simulink model "threeQ_cascaded_relays_real_2024a"  (R2024a)
settings: Solver=VariableStepAuto  StartTime=0.0  StopTime=15  RelTol=1e-3
libraries: spsThreePhaseSeriesRLCLoadLib x2, spsThreePhaseVIMeasurementLib x2, spsThreePhaseBreakerLib x2, spsThreePhaseFaultLib x2, spsDistributedParametersLineLib x1, spsThreePhaseSourceLib x1, spspowerguiLib x1
settings Model: SimulationMode=accelerator  Creator=Carnival  LastModifiedBy=user

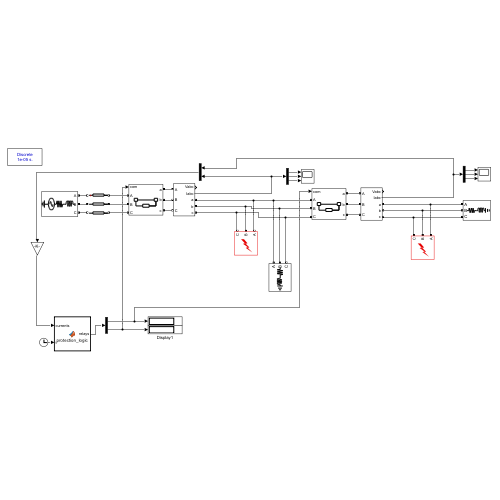
[thumbnail: Simulink's stored preview of the top-level diagram]
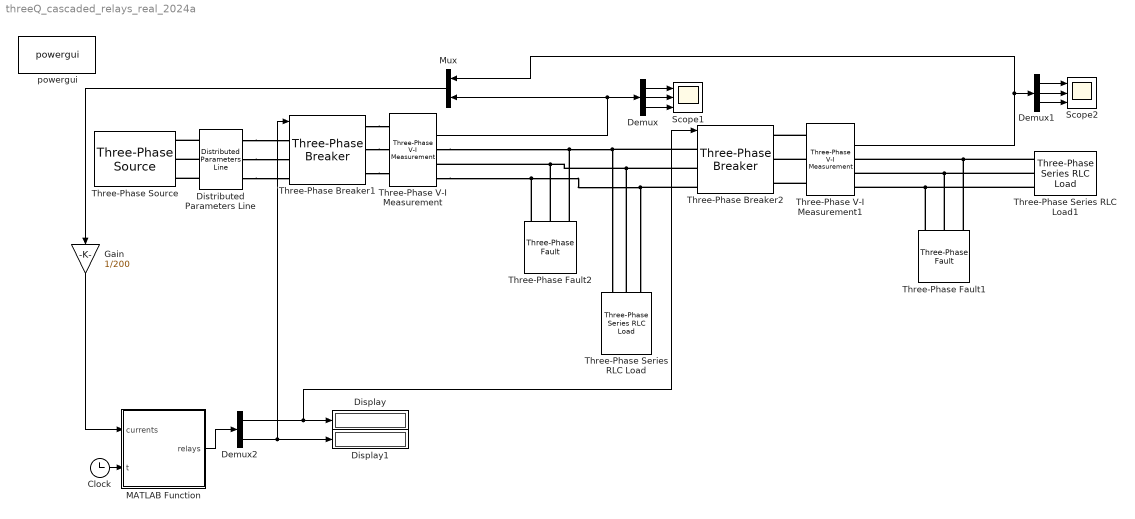
== system threeQ_cascaded_relays_real_2024a ==
  Clock : Clock
  Demux : Demux  Outputs=3
  Demux1 : Demux  Outputs=3
  Demux2 : Demux  Outputs=2
  Display : Display
  Display1 : Display
  Distributed Parameters Line : spsDistributedParametersLineLib/Distributed Parameters Line  Phases=3  Length=15  Frequency=50  Resistance=[0.6273 0.8864]  Inductance="[0.9337e-3  4.1264e-3]"  Capacitance=[12.74e-9 7.751e-9]  x1=[-9e-05 5.02208795910123e-09 1588.76236265853 -8067.37575327395;-8e-05 4.99086976271208e-09 1614.09888914727 -8062.34470644657;-7e-05 4.95960230845327e-09 1639.41948513161 -8057.23408753183;-6e-05 4.92828590492195e-09 1664.72390070749 -8052.04394696949;-5e-05 4.89692086119837e-09 1690.01188613055 -8046.77433598413;-4e-05 4.86550748684287e-09 1715.28319181857 -8041.42530658469;-3e-05 4.83404609189275e-09 1740.53756835399 -8035.99691156393;-2e-05 4.80253698685929e-09 1765.77476648628 -8030.48920449791;-1e-05 4.77098048272463e-09 1790.9945371345 -8024.90223974549]  x2=[-9e-05 4.39159241008057e-08 108.20401185903 -384.846711119618;-8e-05 4.37876771750741e-08 109.412507505629 -384.504879609457;-7e-05 4.36589980826465e-08 110.61992329495 -384.159253191366;-6e-05 4.35298880935337e-08 111.826247310288 -383.809835276536;-5e-05 4.34003484819991e-08 113.03146764571 -383.456629313583;-4e-05 4.32703805265465e-08 114.23557240618 -383.099638788506;-3e-05 4.3139985509907e-08 115.438549707668 -382.738867224658;-2e-05 4.30091647190269e-08 116.640387677276 -382.374318182709;-1e-05 4.28779194450545e-08 117.841074453347 -382.005995260609]  x3=[-9e-05 2.00094431508933e-09 186.56182138791 688.697630075146;-8e-05 2.00283742250668e-09 184.397296886789 689.280331774759;-7e-05 2.00471076272724e-09 182.230952458792 689.856230555771;-6e-05 2.00656431726192e-09 180.062809484864 690.425320734294;-5e-05 2.00839806781686e-09 177.8928893637 690.987596693637;-4e-05 2.0102119962937e-09 175.721213511537 691.543052884364;-3e-05 2.01200608478969e-09 173.547803361938 692.091683824346;-2e-05 2.01378031559791e-09 171.372680365584 692.633484098817;-1e-05 2.0155346712074e-09 169.195865990061 693.168448360428]  x4=[-9e-05 -1.93383320357452e-09 -180.703878471693 -719.166809410987;-8e-05 -1.93593922240759e-09 -178.443661285832 -719.730957511193;-7e-05 -1.9380261343021e-09 -176.181682933075 -720.288002157416;-6e-05 -1.94009391866109e-09 -173.917965738234 -720.837937851849;-5e-05 -1.94214255507634e-09 -171.652532043286 -721.38075916685;-4e-05 -1.94417202332865e-09 -169.385404207145 -721.916460744991;-3e-05 -1.94618230338798e-09 -167.116604605448 -722.445037299114;-2e-05 -1.94817337541369e-09 -164.846155630331 -722.966483612381;-1e-05 -1.95014521975468e-09 -162.57407969021 -723.480794538329]  x5=8.48312350493614e-05  V1=ones(3,3)  V2=ones(3,3)  I1=ones(3,3)  I2=ones(3,3)  nHarmo=1  Measurements=None  Decoupling=off  VsMag0=0  VrMag0=0  VsAngle0=0  VrAngle0=0  IsMag0=0  IrMag0=0  IsAngle0=0  IrAngle0=0
      settings: LibrarySourceBlock=sps_lib/Power Grid Elements/Distributed Parameters Line
  Gain : Gain  Gain=1/200
  MATLAB Function : MATLAB Function  TreatAsAtomicUnit=on
  Mux : Mux  Inputs=2
  Scope1 : Scope  NumInputPorts=3
  Scope2 : Scope  NumInputPorts=3
  Three-Phase Series RLC Load : spsThreePhaseSeriesRLCLoadLib/Three-Phase Series RLC Load  LConnTagsString=A|B|C  Configuration=Y (grounded)  NominalVoltage=11000  Vabc=[1e3 1e3 1e3]  Vabcp=[1e3 1e3 1e3]  NominalFrequency=50  UnbalancedPower=off  ActivePower=2e6  InductivePower=1.2e6  CapacitivePower=0  Pabc=[10e3 9e3 11e3]  QLabc=[100 90 110]  QCabc=[100 90 110]  Pabcp=[10e3 9e3 11e3]  QLabcp=[100 90 110]  QCabcp=[100 90 110]  Measurements=None  LoadType=constant Z
  Three-Phase Series RLC Load1 : spsThreePhaseSeriesRLCLoadLib/Three-Phase Series RLC Load  LConnTagsString=A|B|C  Configuration=Y (grounded)  NominalVoltage=1100  Vabc=[1e3 1e3 1e3]  Vabcp=[1e3 1e3 1e3]  NominalFrequency=50  UnbalancedPower=off  ActivePower=2e6  InductivePower=1.2e6  CapacitivePower=0  Pabc=[10e3 9e3 11e3]  QLabc=[100 90 110]  QCabc=[100 90 110]  Pabcp=[10e3 9e3 11e3]  QLabcp=[100 90 110]  QCabcp=[100 90 110]  Measurements=None  LoadType=constant Z
  Three-Phase V-I Measurement : spsThreePhaseVIMeasurementLib/Three-Phase V-I Measurement  VoltageMeasurement=phase-to-ground  SetLabelV=off  LabelV=Vabc  Vpu=off  VpuLL=off  CurrentMeasurement=yes  SetLabelI=off  LabelI=Iabc  Ipu=off  Pbase=100e6  Vbase=500e3  OutputType=Complex  PhasorSimulation=off  PSBequivalent=0
  Three-Phase V-I Measurement1 : spsThreePhaseVIMeasurementLib/Three-Phase V-I Measurement  VoltageMeasurement=phase-to-ground  SetLabelV=off  LabelV=Vabc  Vpu=off  VpuLL=off  CurrentMeasurement=yes  SetLabelI=off  LabelI=Iabc  Ipu=off  Pbase=100e6  Vbase=500e3  OutputType=Complex  PhasorSimulation=off  PSBequivalent=0
  Three-Phase Breaker1 : spsThreePhaseBreakerLib/Three-Phase Breaker  InitialState=closed  SwitchA=on  SwitchB=on  SwitchC=on  SwitchTimes="[1/60  5/60]"  External=on  BreakerResistance=0.01  SnubberResistance=1e6  SnubberCapacitance=inf  Measurements=None
  Three-Phase Breaker2 : spsThreePhaseBreakerLib/Three-Phase Breaker  InitialState=closed  SwitchA=on  SwitchB=on  SwitchC=on  SwitchTimes="[1/60  5/60]"  External=on  BreakerResistance=0.01  SnubberResistance=1e6  SnubberCapacitance=inf  Measurements=None
  Three-Phase Fault1 : spsThreePhaseFaultLib/Three-Phase Fault  InitialStates=0  FaultA=off  FaultB=on  FaultC=on  GroundFault=on  SwitchTimes="[5  6]"  External=off  SwitchStatus=NaN  FaultResistance=0.001  GroundResistance=0.01  SnubberResistance=1e6  SnubberCapacitance=inf  Measurements=None
  Three-Phase Fault2 : spsThreePhaseFaultLib/Three-Phase Fault  InitialStates=0  FaultA=off  FaultB=on  FaultC=on  GroundFault=off  SwitchTimes="[5  6]"  External=off  SwitchStatus=NaN  FaultResistance=0.001  GroundResistance=0.01  SnubberResistance=1e6  SnubberCapacitance=inf  Measurements=None
  Three-Phase Source : spsThreePhaseSourceLib/Three-Phase Source  InternalConnection=Yg  VoltagePhases=off  Voltage=11000  PhaseAngle=0  Voltage_phases=[25e3 25e3 25e3]/sqrt(3)  PhaseAngles_phases=[0 -120 +120]  Frequency=50  NonIdealSource=on  SpecifyImpedance=off  Resistance=0.8929  Inductance=16.58e-3  ShortCircuitLevel=100e6  BaseVoltage=11000  XRratio=7  BusType=swing  Pref=10e3  Qref=0  Prefabc=[10e3, 10e3, 10e3]  Qrefabc=[0, 0, 0]  Qmin=-inf  Qmax=inf
  powergui : spspowerguiLib/powergui  Priority=1  SimulationMode=Discrete  SampleTime=1e-5  frequency=60  Iterations=50  frequencyindice=0  Pbase=100e6  ErrMax=1e-4  UnitsV=kV  UnitsW=MW  buscounter=0  FunctionMessages=off  echomessages=off  EnableUseOfTLC=off  CurrentSourceSwitches=off  DisableSnubberDevices=off  DisableRonSwitches=off  DisableVfSwitches=off  DisplayEquations=off  AutomaticDiscreteSolvers=off  SolverType=Tustin/Backward Euler (TBE)  Interpol=off  ExternalGateDelay=off  methode=off  Ts=100  x0status=blocks  SPID=on  SwTol=0  HookPort=off  NonlinearTolerance=1e-4  nMaxIteration=100  ContinueOnMaxIteration=off  RestoreLinks=warning  ResistiveCurrentMeasurement=off  Frange=[0:2:500]  Ylog=off  Xlog=on  ShowGrid=off  save=off  variable=ZData  structure=0  ZoomFFT=off  StartTime=0.0  cycles=1  DisplayStyle=1  fundamental=60  FreqAxis=off  MaxFrequency=1000  frequencyindicesteady=1  RmsSteady=1  display=off
  wires:
  Three-Phase V-I Measurement/2 -> Mux/2, Demux/1
  Three-Phase V-I Measurement1/2 -> Mux/1, Demux1/1
  Demux/1 -> Scope1/1
  Demux/2 -> Scope1/2
  Demux/3 -> Scope1/3
  Demux1/1 -> Scope2/1
  Demux1/2 -> Scope2/2
  Demux1/3 -> Scope2/3
  Clock/1 -> MATLAB Function/2(t)
  Demux2/1 -> Display/1, Three-Phase Breaker2/1
  Mux/1 -> Gain/1
  Gain/1 -> MATLAB Function/1(currents)
  MATLAB Function/1(relays) -> Demux2/1
  Demux2/2 -> Display1/1, Three-Phase Breaker1/1
  connections:
  Three-Phase Breaker1/RConn1 -- Three-Phase V-I Measurement/LConn1
  Three-Phase Breaker1/RConn2 -- Three-Phase V-I Measurement/LConn2
  Three-Phase Breaker1/RConn3 -- Three-Phase V-I Measurement/LConn3
  Three-Phase V-I Measurement/RConn1 -- Three-Phase Fault2/LConn1 -- Three-Phase Breaker2/LConn1 -- Three-Phase Series RLC Load/LConn1
  Three-Phase Series RLC Load/LConn2 -- Three-Phase V-I Measurement/RConn2 -- Three-Phase Fault2/LConn2 -- Three-Phase Breaker2/LConn2
  Three-Phase V-I Measurement/RConn3 -- Three-Phase Fault2/LConn3 -- Three-Phase Breaker2/LConn3 -- Three-Phase Series RLC Load/LConn3
  Three-Phase V-I Measurement1/LConn1 -- Three-Phase Breaker2/RConn1
  Three-Phase V-I Measurement1/LConn2 -- Three-Phase Breaker2/RConn2
  Three-Phase V-I Measurement1/LConn3 -- Three-Phase Breaker2/RConn3
  Three-Phase Series RLC Load1/LConn3 -- Three-Phase Fault1/LConn3 -- Three-Phase V-I Measurement1/RConn3
  Three-Phase Series RLC Load1/LConn2 -- Three-Phase Fault1/LConn2 -- Three-Phase V-I Measurement1/RConn2
  Three-Phase Series RLC Load1/LConn1 -- Three-Phase Fault1/LConn1 -- Three-Phase V-I Measurement1/RConn1
  Distributed Parameters Line/LConn2 -- Three-Phase Source/RConn2
  Distributed Parameters Line/LConn3 -- Three-Phase Source/RConn3
  Distributed Parameters Line/LConn1 -- Three-Phase Source/RConn1
  Distributed Parameters Line/RConn1 -- Three-Phase Breaker1/LConn1
  Distributed Parameters Line/RConn2 -- Three-Phase Breaker1/LConn2
  Distributed Parameters Line/RConn3 -- Three-Phase Breaker1/LConn3

== matlab function threeQ_cascaded_relays_real_2024a/MATLAB Function ==
  settings: updateMethod=DISCRETE
  data: currents input; relays output; t input
function relays = protection_logic(currents, t)

%% =========================================================
% PROFESSIONAL IDMT CASCADED OVERCURRENT RELAY
% 11 kV Egyptian Distribution Feeder
%% =========================================================

%% OUTPUT
relays = [1;1];

%% =========================================================
%% PERSISTENT VARIABLES
%% =========================================================

persistent t_pick1 t_pick2
persistent picked1 picked2
persistent trip1 trip2
persistent t_trip1 t_trip2

if isempty(picked1)

    picked1 = false;
    picked2 = false;

    trip1 = false;
    trip2 = false;

    t_pick1 = 0;
    t_pick2 = 0;

    t_trip1 = -inf;
    t_trip2 = -inf;

end

%% =========================================================
%% RELAY SETTINGS
%% =========================================================

% =========================================================
% REALISTIC 11 kV FEEDER SETTINGS
% =========================================================

% Pickup current (Amperes)
I_pickup = 350;

% IEC Standard Inverse
K = 0.14;
alpha = 0.02;

% Time multiplier settings
TMS1 = 0.20;    % upstream
TMS2 = 0.05;    % downstream

% Reset memory
reset_time = 0.20;

% Backup delay
backup_delay = 0.30;

%% =========================================================
%% CURRENT EXTRACTION
%% currents = [Ia1 Ib1 Ic1 Ia2 Ib2 Ic2]
%% =========================================================

vals = abs(currents(:)');

Ia1 = vals(1);
Ib1 = vals(2);
Ic1 = vals(3);

Ia2 = vals(4);
Ib2 = vals(5);
Ic2 = vals(6);

max1 = max([Ia1 Ib1 Ic1]);
max2 = max([Ia2 Ib2 Ic2]);

%% =========================================================
%% PICKUP LOGIC
%% =========================================================

% ---------------------------------------------------------
% DOWNSTREAM RELAY
% ---------------------------------------------------------

if max2 > I_pickup

    if ~picked2
        picked2 = true;
        t_pick2 = t;
    end

else

    if (t - t_pick2) > reset_time
        picked2 = false;
    end

end

% ---------------------------------------------------------
% UPSTREAM RELAY
% ---------------------------------------------------------

if max1 > I_pickup

    if ~picked1
        picked1 = true;
        t_pick1 = t;
    end

else

    if (t - t_pick1) > reset_time
        picked1 = false;
    end

end

%% =========================================================
%% IDMT OPERATING TIME
%% =========================================================

tripDelay1 = inf;
tripDelay2 = inf;

% ---------------------------------------------------------
% DOWNSTREAM
% ---------------------------------------------------------

if picked2

    ratio2 = max2 / I_pickup;

    if ratio2 <= 1
        ratio2 = 1.001;
    end

    tripDelay2 = (K*TMS2) / ((ratio2^alpha) - 1);

end

% ---------------------------------------------------------
% UPSTREAM
% ---------------------------------------------------------

if picked1

    ratio1 = max1 / I_pickup;

    if ratio1 <= 1
        ratio1 = 1.001;
    end

    tripDelay1 = (K*TMS1) / ((ratio1^alpha) - 1);

end

%% =========================================================
%% TRIP LOGIC
%% =========================================================

% ---------------------------------------------------------
% DOWNSTREAM RELAY TRIPS FIRST
% ---------------------------------------------------------

if picked2 && ~trip2

    if (t - t_pick2) >= tripDelay2

        trip2 = true;
        t_trip2 = t;

    end

end

% ---------------------------------------------------------
% UPSTREAM RELAY
% ---------------------------------------------------------

if picked1 && ~trip1

    % coordination blocking
    if ~trip2

        if (t - t_pick1) >= tripDelay1

            trip1 = true;
            t_trip1 = t;

        end

    end

end

%% =========================================================
%% BACKUP PROTECTION
%% =========================================================

if picked1 && trip2 && ~trip1

    if (t - t_trip2) >= backup_delay

        trip1 = true;
        t_trip1 = t;

    end

end

%% =========================================================
%% OUTPUTS
%% 1 = CLOSED
%% 0 = OPEN
%% =========================================================

relays(1) = double(~trip1);
relays(2) = double(~trip2);

end
